simulink model "Chilis1"  (R2024a)
settings: Solver=VariableStepAuto  StartTime=0.0  StopTime=10.0  RelTol=1e-3
settings Model: Creator=rapha  LastModifiedBy=rapha

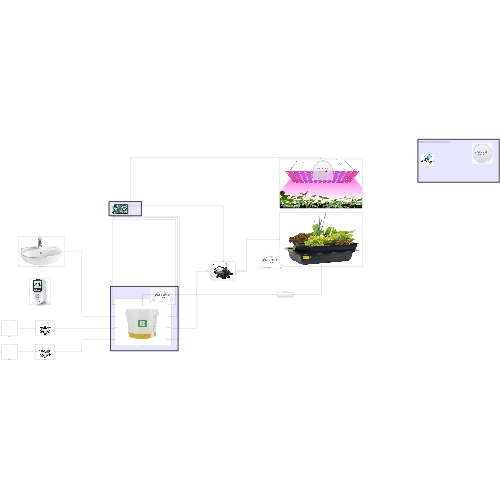
[thumbnail: Simulink's stored preview of the top-level diagram]
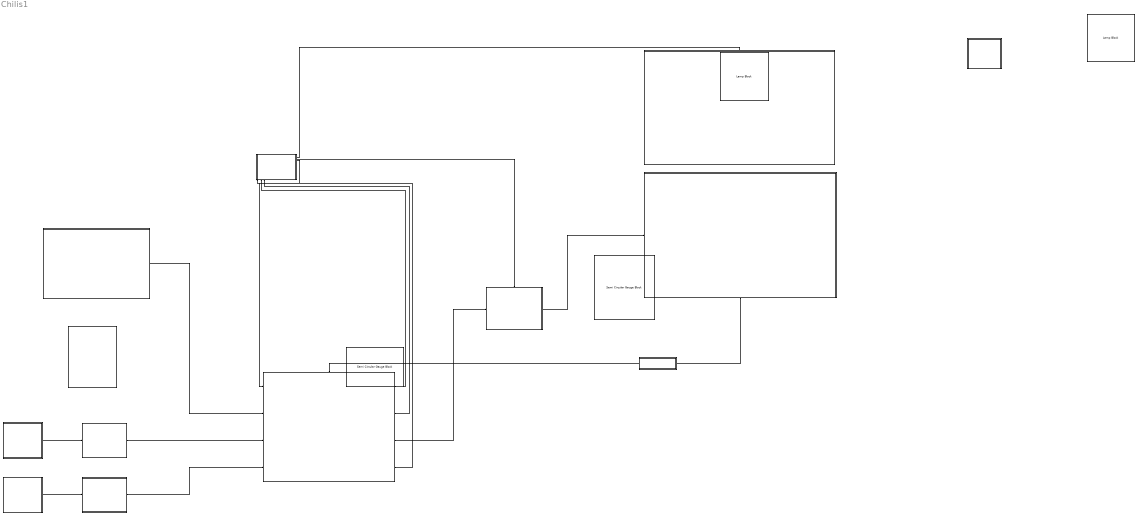
== system Chilis1 ==
  note: Steuerung
  note: Dashboard
      |
      | Hygrometer (Verdunstung und Darmstadt Temperaturen), Water-Leakage, Füllstände,
      | Wasserauffüll monitoring, Stromverbrauch, Pflanzen wachstum, Licht Regelung
  Arduino : Subsystem
      settings: PortSchema="{\"entries\":[{\"content\":{\"sides\":[{\"content\":{},\"type\":\"ConnectorPlacement.EquallySpacedRectSide\",\"uuid\":\"3b6a8aa3-f5f4-4eae-beef-162476917ea7\"},{\"content\":{\"connectorIds\":[\"Out1\",\"Out2\",\"Out3\",\"Out4\",\"Out5\",\"Out6\",\"Out7\",\"Out8\",\"Out9\",\"Out10\",\"Out11\",\"Out12\"],\"side\":\"RIGHT\"},\"type\":\"ConnectorPlacement.EquallySpacedRectSide\",\"uuid\":\"3e057b3c-23fd-4663-9ff4-7029424d3a96\"},{\"content\":{\"side\":\"TOP\"},\"type\":\"ConnectorPlacement.EquallySpacedRectSide\",\"uuid\":\"2f6ad2ff-0ad1-48cc-bb1f-ada745819d57\"},{\"content\":{\"connectorIds\":[\"In1\",\"In2\",\"In3\",\"In4\",\"In5\",\"In6\",\"In7\",\"In8\",\"In9\",\"In10\",\"In11\",\"In12\"],\"side\":\"BOTTOM\"},\"type\":\"ConnectorPlacement.EquallySpacedRectSide\",\"uuid\":\"df01ff17-dde7-40e9-ab93-85a34753e43a\"}]},\"type\":\"ConnectorPlacement.EquallySpacedConnector\",\"uuid\":\"05ef216b-003e-4d9c-aa01-62d58e57fe93\"}],\"packageUris\":[\"http://schema.mathworks.com/mf0/Connector/R2020b\"],\"version\":\"1.0\"}"
      mask Display: image('Herunterladen.jpeg');
  Arduino1 : Subsystem
      mask Display: image('Hygrometer.jpeg');
  Arduino2 : Subsystem
      mask Display: image('Peristaltik Pumpe.jpg');
  Arduino4 : Subsystem
      mask Display: text(5, 10, 'PH -','FontSize',20);
  Arduino6 : Subsystem
      mask Display: image('Peristaltik Pumpe.jpg');
  Arduino7 : Subsystem
      mask Display: text(5, 10, 'PH -','FontSize',20);
  Half Gauge : SemiCircularGaugeBlock
  Half Gauge1 : SemiCircularGaugeBlock
  Lamp : LampBlock  LabelPosition=Hide
  Lamp1 : LampBlock  LabelPosition=Hide
  Stromzäler und Qulle : Subsystem
      mask Display: image('Stromzähler.jpeg');
  Stromzäler und Qulle1 : Subsystem
      mask Display: image('Waschbecken.jpeg');
  Subsystem : Subsystem
      settings: PortSchema="{\"entries\":[{\"content\":{\"sides\":[{\"content\":{\"connectorIds\":[\"In1\",\"In2\",\"In3\",\"In4\"]},\"type\":\"ConnectorPlacement.EquallySpacedRectSide\",\"uuid\":\"5f2b13a7-e349-4945-a47b-b355f0493e96\"},{\"content\":{\"connectorIds\":[\"Out1\",\"Out2\",\"Out3\",\"Out4\"],\"side\":\"RIGHT\"},\"type\":\"ConnectorPlacement.EquallySpacedRectSide\",\"uuid\":\"ed74b2c3-73b7-4395-be98-8863f2462565\"},{\"content\":{\"connectorIds\":[\"In5\"],\"side\":\"TOP\"},\"type\":\"ConnectorPlacement.EquallySpacedRectSide\",\"uuid\":\"457c3599-37f7-42b0-98f6-5a6db61e721d\"}]},\"type\":\"ConnectorPlacement.EquallySpacedConnector\",\"uuid\":\"c8d1bd34-1cf4-47ae-898c-ae362d6606b0\"}],\"packageUris\":[\"http://schema.mathworks.com/mf0/Connector/R2020b\"],\"version\":\"1.0\"}"
      mask Display: image('Eimer.jpg');
  Subsystem1 : Subsystem
      settings: PortSchema="{\"entries\":[{\"content\":{\"sides\":[{\"content\":{\"connectorIds\":[\"In1\"]},\"type\":\"ConnectorPlacement.EquallySpacedRectSide\",\"uuid\":\"3b6a8aa3-f5f4-4eae-beef-162476917ea7\"},{\"content\":{\"side\":\"RIGHT\"},\"type\":\"ConnectorPlacement.EquallySpacedRectSide\",\"uuid\":\"3e057b3c-23fd-4663-9ff4-7029424d3a96\"},{\"content\":{\"side\":\"TOP\"},\"type\":\"ConnectorPlacement.EquallySpacedRectSide\",\"uuid\":\"2f6ad2ff-0ad1-48cc-bb1f-ada745819d57\"},{\"content\":{\"connectorIds\":[\"Out1\"],\"side\":\"BOTTOM\"},\"type\":\"ConnectorPlacement.EquallySpacedRectSide\",\"uuid\":\"d96ac3e7-64b0-4b25-916e-fd71b97ae106\"}]},\"type\":\"ConnectorPlacement.EquallySpacedConnector\",\"uuid\":\"05ef216b-003e-4d9c-aa01-62d58e57fe93\"}],\"packageUris\":[\"http://schema.mathworks.com/mf0/Connector/R2020b\"],\"version\":\"1.0\"}"
      mask Display: image('Flutbecken.jpeg');
  Subsystem2 : Subsystem
      settings: PortSchema="{\"entries\":[{\"content\":{\"sides\":[{\"content\":{\"connectorIds\":[\"In1\"]},\"type\":\"ConnectorPlacement.EquallySpacedRectSide\",\"uuid\":\"161a8875-b57f-49fc-8019-866a443a3fdf\"},{\"content\":{\"connectorIds\":[\"Out1\"],\"side\":\"RIGHT\"},\"type\":\"ConnectorPlacement.EquallySpacedRectSide\",\"uuid\":\"abe0a26c-fd1c-4a74-98d9-01c0287a807a\"},{\"content\":{\"connectorIds\":[\"In2\"],\"side\":\"TOP\"},\"type\":\"ConnectorPlacement.EquallySpacedRectSide\",\"uuid\":\"eea1c959-2ba6-4798-854f-e0c11a7f36b0\"}]},\"type\":\"ConnectorPlacement.EquallySpacedConnector\",\"uuid\":\"cb602760-7f2c-43eb-a6fb-673c5802800a\"}],\"packageUris\":[\"http://schema.mathworks.com/mf0/Connector/R2020b\"],\"version\":\"1.0\"}"
      mask Display: image('Lichter.jpg');
  Subsystem3 : Subsystem
      settings: PortSchema="{\"entries\":[{\"content\":{\"sides\":[{\"content\":{\"connectorIds\":[\"In1\"]},\"type\":\"ConnectorPlacement.EquallySpacedRectSide\",\"uuid\":\"161a8875-b57f-49fc-8019-866a443a3fdf\"},{\"content\":{\"connectorIds\":[\"Out1\"],\"side\":\"RIGHT\"},\"type\":\"ConnectorPlacement.EquallySpacedRectSide\",\"uuid\":\"abe0a26c-fd1c-4a74-98d9-01c0287a807a\"},{\"content\":{\"connectorIds\":[\"In2\"],\"side\":\"TOP\"},\"type\":\"ConnectorPlacement.EquallySpacedRectSide\",\"uuid\":\"eea1c959-2ba6-4798-854f-e0c11a7f36b0\"}]},\"type\":\"ConnectorPlacement.EquallySpacedConnector\",\"uuid\":\"cb602760-7f2c-43eb-a6fb-673c5802800a\"}],\"packageUris\":[\"http://schema.mathworks.com/mf0/Connector/R2020b\"],\"version\":\"1.0\"}"
      mask Display: image('Pumpe.jpeg');
  Verdunstung : Subsystem
  wires:
  Subsystem/3(Wasserstand) -> Subsystem3/1(In1)  "Waasergemisch"
  Subsystem3/1(Out1) -> Subsystem1/1(In1)  "Pflanzen Zufluss (Flut Richtung)"
  Stromzäler und Qulle1/1(Out1) -> Subsystem/2(Auffülllen)
  Subsystem1/1(Out1) -> Verdunstung/1(In1)
  Arduino6/1(Out1) -> Subsystem/3(Minerallösung)
  Arduino2/1(Out1) -> Subsystem/4(PH +)
  Arduino7/1(Out1) -> Arduino6/1(In1)
  Verdunstung/1(Out1) -> Subsystem/5(Pflanzen Rückfluss (Ebbe))
  Arduino4/1(Out1) -> Arduino2/1(In1)
  Subsystem/1(EC Wert) -> Arduino/2(In2)
  Subsystem/2(PH Wert) -> Arduino/3(In3)
  Subsystem/4(Wassertemperatur) -> Arduino/1(In1)
  Arduino/2(Out2) -> Subsystem3/2(In2)
  Arduino/1(Out1) -> Subsystem2/2(In1)
  Arduino/3(Out3) -> Subsystem/1(Rührer ein)

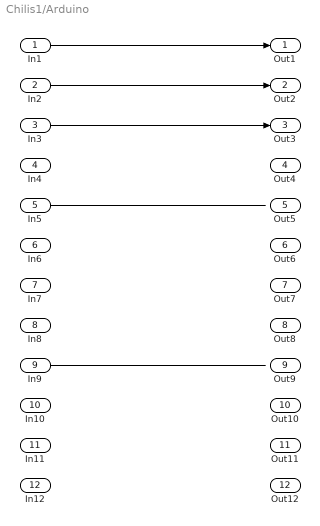
== system Chilis1/Arduino ==
  In1 : Inport
  In2 : Inport  Port=2
  In3 : Inport  Port=3
  In4 : Inport  Port=4
  In5 : Inport  Port=5
  In6 : Inport  Port=6
  In7 : Inport  Port=7
  In8 : Inport  Port=8
  In9 : Inport  Port=9
  In10 : Inport  Port=10
  In11 : Inport  Port=11
  In12 : Inport  Port=12
  Out1 : Outport
  Out2 : Outport  Port=2
  Out3 : Outport  Port=3
  Out4 : Outport  Port=4
  Out5 : Outport  Port=5
  Out6 : Outport  Port=6
  Out7 : Outport  Port=7
  Out8 : Outport  Port=8
  Out9 : Outport  Port=9
  Out10 : Outport  Port=10
  Out11 : Outport  Port=11
  Out12 : Outport  Port=12
  wires:
  In1/1 -> Out1/1
  In5/1 -> ?
  In9/1 -> ?
  In2/1 -> Out2/1
  In3/1 -> Out3/1

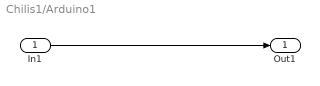
== system Chilis1/Arduino1 ==
  In1 : Inport
  Out1 : Outport
  wires:
  In1/1 -> Out1/1

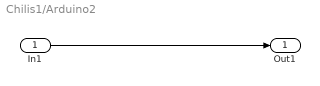
== system Chilis1/Arduino2 ==
  In1 : Inport
  Out1 : Outport
  wires:
  In1/1 -> Out1/1

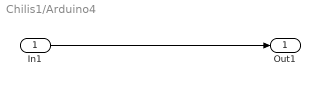
== system Chilis1/Arduino4 ==
  In1 : Inport
  Out1 : Outport
  wires:
  In1/1 -> Out1/1

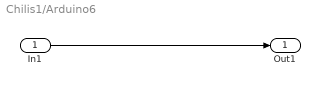
== system Chilis1/Arduino6 ==
  In1 : Inport
  Out1 : Outport
  wires:
  In1/1 -> Out1/1

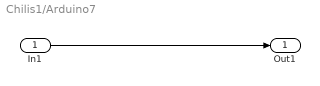
== system Chilis1/Arduino7 ==
  In1 : Inport
  Out1 : Outport
  wires:
  In1/1 -> Out1/1

== system Chilis1/Stromzäler und Qulle ==
  In1 : Inport
  Out1 : Outport
  wires:
  In1/1 -> Out1/1

== system Chilis1/Stromzäler und Qulle1 ==
  In1 : Inport
  Out1 : Outport
  wires:
  In1/1 -> Out1/1

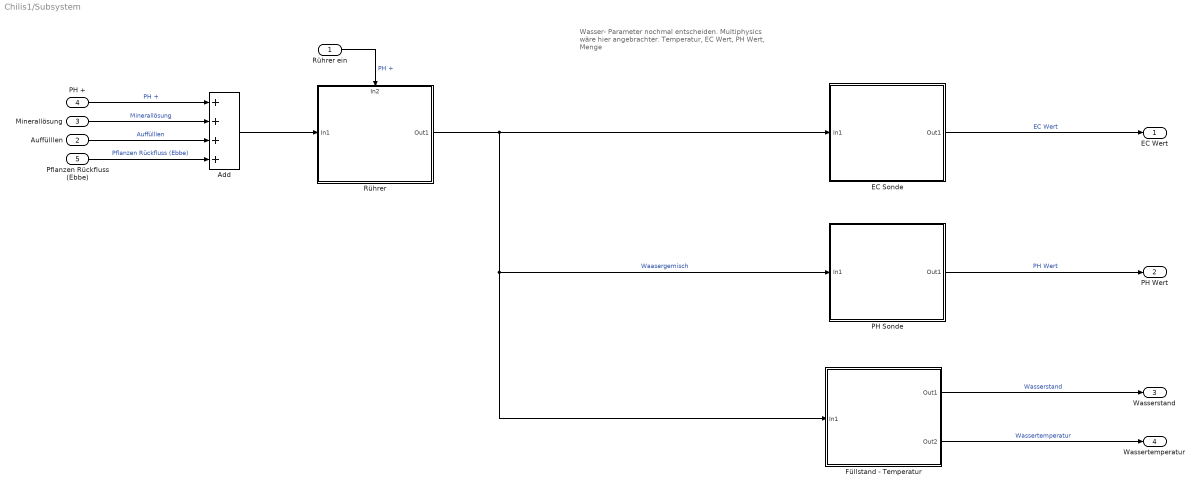
== system Chilis1/Subsystem ==
  note: Wasser- Parameter nochmal entscheiden.
      |
      | Multiphysics wäre hier angebrachter.
      |
      | Temperatur, EC Wert, PH Wert,
      | Menge
  Rührer ein : Inport
  Auffülllen : Inport  Port=2
  Minerallösung : Inport  Port=3
  PH + : Inport  Port=4
  Pflanzen Rückfluss (Ebbe) : Inport  Port=5
  Add : Sum  Inputs=++++
  EC Sonde : Subsystem
      mask Display: image('EC Meter.jpeg');
  Füllstand - Temperatur : Subsystem
      mask Display: text(40, 60, ['Wasserstand \n      und \n Temperatur']);
  PH Sonde : Subsystem
      mask Display: image('PH Sonde.jpg');
  Rührer : Subsystem
      settings: PortSchema="{\"entries\":[{\"content\":{\"sides\":[{\"content\":{\"connectorIds\":[\"In1\"]},\"type\":\"ConnectorPlacement.EquallySpacedRectSide\",\"uuid\":\"161a8875-b57f-49fc-8019-866a443a3fdf\"},{\"content\":{\"connectorIds\":[\"Out1\"],\"side\":\"RIGHT\"},\"type\":\"ConnectorPlacement.EquallySpacedRectSide\",\"uuid\":\"abe0a26c-fd1c-4a74-98d9-01c0287a807a\"},{\"content\":{\"connectorIds\":[\"In2\"],\"side\":\"TOP\"},\"type\":\"ConnectorPlacement.EquallySpacedRectSide\",\"uuid\":\"eea1c959-2ba6-4798-854f-e0c11a7f36b0\"}]},\"type\":\"ConnectorPlacement.EquallySpacedConnector\",\"uuid\":\"cb602760-7f2c-43eb-a6fb-673c5802800a\"}],\"packageUris\":[\"http://schema.mathworks.com/mf0/Connector/R2020b\"],\"version\":\"1.0\"}"
      mask Display: image('Rührer.png');
  EC Wert : Outport
  PH Wert : Outport  Port=2
  Wasserstand : Outport  Port=3
  Wassertemperatur : Outport  Port=4
  wires:
  EC Sonde/1(Out1) -> EC Wert/1  "EC Wert"
  PH Sonde/1(Out1) -> PH Wert/1  "PH Wert"
  Rührer/1(Out1) -> PH Sonde/1(In1), Füllstand - Temperatur/1(In1), EC Sonde/1(In1)  "Waasergemisch"
  Füllstand - Temperatur/1(Out1) -> Wasserstand/1  "Wasserstand"
  Auffülllen/1 -> Add/3  "Auffülllen"
  Pflanzen Rückfluss (Ebbe)/1 -> Add/4  "Pflanzen Rückfluss (Ebbe)"
  Minerallösung/1 -> Add/2  "Minerallösung"
  PH +/1 -> Add/1  "PH +"
  Add/1 -> Rührer/1(In1)
  Füllstand - Temperatur/2(Out2) -> Wassertemperatur/1  "Wassertemperatur"
  Rührer ein/1 -> Rührer/2(In2)  "PH +"

== system Chilis1/Subsystem1 ==
  In1 : Inport
  Out1 : Outport
  wires:
  In1/1 -> Out1/1

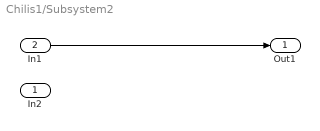
== system Chilis1/Subsystem2 ==
  In2 : Inport
  In1 : Inport  Port=2
  Out1 : Outport
  wires:
  In1/1 -> Out1/1

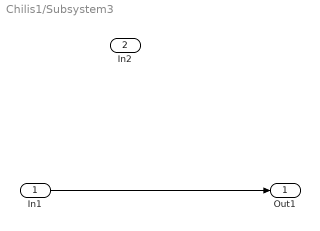
== system Chilis1/Subsystem3 ==
  In1 : Inport
  In2 : Inport  Port=2
  Out1 : Outport
  wires:
  In1/1 -> Out1/1

== system Chilis1/Verdunstung ==
  In1 : Inport
  Out1 : Outport
  wires:
  In1/1 -> Out1/1

== system Chilis1/Subsystem/EC Sonde ==
  In1 : Inport
  Out1 : Outport
  wires:
  In1/1 -> Out1/1

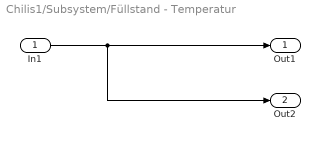
== system Chilis1/Subsystem/Füllstand - Temperatur ==
  In1 : Inport
  Out1 : Outport
  Out2 : Outport  Port=2
  wires:
  In1/1 -> Out2/1, Out1/1

== system Chilis1/Subsystem/PH Sonde ==
  In1 : Inport
  Out1 : Outport
  wires:
  In1/1 -> Out1/1

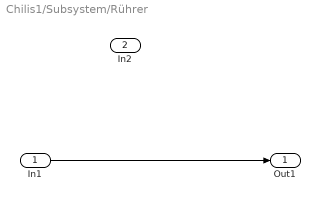
== system Chilis1/Subsystem/Rührer ==
  In1 : Inport
  In2 : Inport  Port=2
  Out1 : Outport
  wires:
  In1/1 -> Out1/1
